simulink model "test"  (R2018b)
settings: Solver=VariableStepAuto  StartTime=0.0  StopTime=1  RelTol=1e-3
settings Model: Creator=Admin  LastModifiedBy=Admin
settings DataIOCC: SaveFormat=Array  SaveTime=off

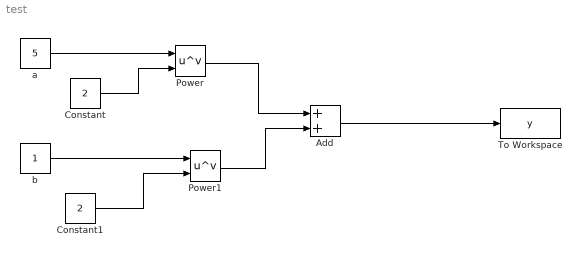
== system test ==
  Add : Sum
  Constant : Constant  Value=2
  Constant1 : Constant  Value=2
  Power : Math  Operator=pow  SaturateOnIntegerOverflow=on
  Power1 : Math  Operator=pow  SaturateOnIntegerOverflow=on
  To Workspace : ToWorkspace  VariableName=y  SampleTime=-1
  a : Constant  Value=5
  b : Constant
  wires:
  Add/1 -> To Workspace/1
  Constant1/1 -> Power1/2
  b/1 -> Power1/1
  Constant/1 -> Power/2
  a/1 -> Power/1
  Power/1 -> Add/1
  Power1/1 -> Add/2
